simulink library "dual_RL_load"  (R2025b)
settings: Solver=VariableStepAuto  StartTime=0.0  StopTime=10.0  RelTol=1e-3
libraries: fl_lib x9
settings Model: Creator=ltnbda  LastModifiedBy=ltnbda

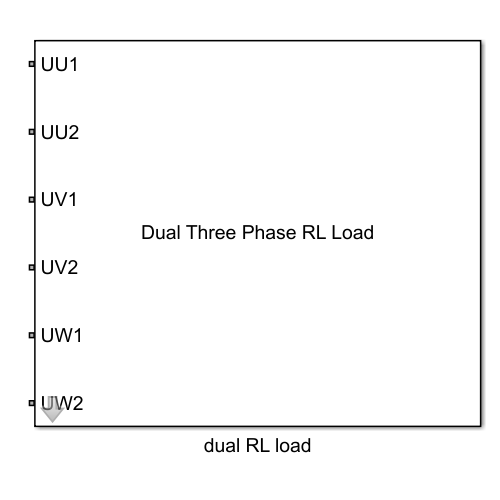
[thumbnail: Simulink's stored preview of the top-level diagram]
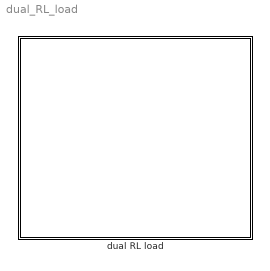
== system dual_RL_load ==
  dual RL load : Subsystem  mask{Ls_load=1e-3, Rs_load=1}
      mask prompts: Ls_load "Ls_load (H)"; Rs_load "Rs_load (Ohm)"
      mask Display:
      | disp('Dual Three Phase RL Load');
      | port_label('lconn', 1, 'UU1');
      | port_label('lconn', 2, 'UU2');
      | port_label('lconn', 3, 'UV1');
      | port_label('lconn', 4, 'UV2');
      | port_label('lconn', 5, 'UW1');
      | port_label('lconn', 6, 'UW2');

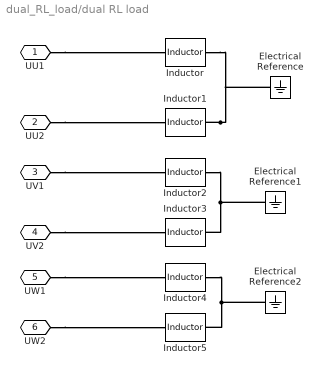
== system dual_RL_load/dual RL load ==
  Electrical Reference : fl_lib/Electrical/Electrical Elements/Electrical Reference
  Electrical Reference1 : fl_lib/Electrical/Electrical Elements/Electrical Reference
  Electrical Reference2 : fl_lib/Electrical/Electrical Elements/Electrical Reference
  Inductor{,1..5} (6 alike) : fl_lib/Electrical/Electrical Elements/Inductor  l=Ls_load H  r=Rs_load Ohm  g=1e-9 1/Ohm  i_specify=off  i_priority=None  i=0 A  i_nominal_specify=off  i_nominal_value=1  i_nominal_unit=A  v_specify=off  v_priority=None  v=0 V  v_nominal_specify=off  v_nominal_value=1  v_nominal_unit=V  i_L_specify=off  i_L_priority=High  i_L=0 A  i_L_nominal_specify=off  i_L_nominal_value=1  i_L_nominal_unit=A
  UU1 : PMIOPort  Side=Left
  UU2 : PMIOPort  Port=2  Side=Left
  UV1 : PMIOPort  Port=3  Side=Left
  UV2 : PMIOPort  Port=4  Side=Left
  UW1 : PMIOPort  Port=5  Side=Left
  UW2 : PMIOPort  Port=6  Side=Left
  connections:
  Inductor2/RConn1 -- Electrical Reference1/LConn1 -- Inductor3/RConn1
  Inductor4/RConn1 -- Electrical Reference2/LConn1 -- Inductor5/RConn1
  UV2/RConn1 -- Inductor3/LConn1
  Inductor1/RConn1 -- Inductor/RConn1 -- Electrical Reference/LConn1
  UU1/RConn1 -- Inductor/LConn1
  UW2/RConn1 -- Inductor5/LConn1
  UU2/RConn1 -- Inductor1/LConn1
  UW1/RConn1 -- Inductor4/LConn1
  UV1/RConn1 -- Inductor2/LConn1
